simulink model "regolatore_P_Bias"  (R2018a)
settings: Solver=FixedStepAuto  StartTime=0.0  StopTime=8000  RelTol=1e-3
undefined symbols (not defined in the file or in its folder): kP
libraries: cstblocks x1
settings Model: Creator=peppe  LastModifiedBy=peppe

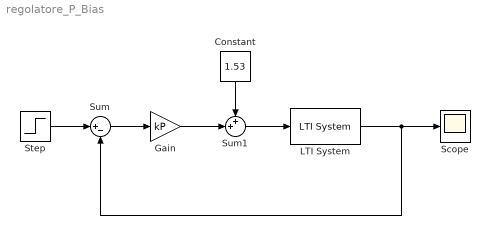
== system regolatore_P_Bias ==
  Constant : Constant  Value=1.53
  Gain : Gain  Gain=kP
  LTI System : cstblocks/LTI System  sys=G  IC=[]
  Scope : Scope
  Step : Step  SampleTime=0
  Sum : Sum  Inputs=|+-
  Sum1 : Sum  Inputs=++|
  wires:
  Step/1 -> Sum/1
  Sum/1 -> Gain/1
  Gain/1 -> Sum1/2
  Constant/1 -> Sum1/1
  Sum1/1 -> LTI System/1
  LTI System/1 -> Sum/2, Scope/1
